simulink model "OREGO"  (Simulink 10.0)
settings: Solver=ode45  StartTime=0.0  StopTime=360  RelTol=1e-3  EnableMultiTasking=on
settings Model: Creator=UX31  LastModifiedBy=unknown
settings DataIOCC: LimitDataPoints=on
settings DebuggingCC: UnderspecifiedInitializationDetection=Simplified  MergeDetectMultiDrivingBlocksExec=error  SolverPrmCheckMsg=warning
settings GRTTargetCC: GeneratePreprocessorConditionals=Disable all  CombineOutputUpdateFcns=on  GRTInterface=off
settings ConfigComp: CovExternalEMLEnable=off  CovSFcnEnable=off

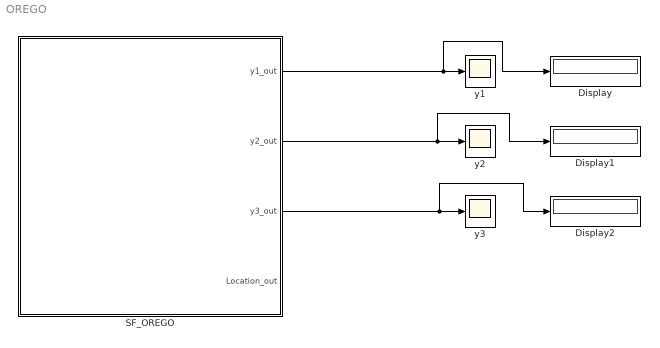
== system OREGO ==
  Display : Display
  Display1 : Display
  Display2 : Display
  SF_OREGO : Stateflow chart  TreatAsAtomicUnit=on
  y1 : Scope
  y2 : Scope
  y3 : Scope
  wires:
  SF_OREGO/1(y1_out) -> Display/1, y1/1
  SF_OREGO/2(y2_out) -> Display1/1, y2/1
  SF_OREGO/3(y3_out) -> Display2/1, y3/1

== stateflow chart SF_OREGO ==
  settings: updateMethod=CONTINUOUS
  state OREGO
    du:
    y1_dot=s*(y2-y1*y2+y1-q*y1^2);
    y2_dot=(1/s)*(0-y2-y1*y2+y3);
    y3_dot=w*(y1-y3);
    y1_out=y1;
    y2_out=y2;
    y3_out=y3;
    Location_out =1;
  (default) -> OREGO : {y1=1;y2=2;y3=3}
  data: y1 local double; y1_out output double; y2 local double; y2_out output double; y3 local double; y3_out output double; Location_out output double; s constant double =77.27; q constant double =8.375*10^-6; w constant double =0.161
  data y1 settings: updateMethod=SF_CONTINUOUS_TIME_DATA
  data y2 settings: updateMethod=SF_CONTINUOUS_TIME_DATA
  data y3 settings: updateMethod=SF_CONTINUOUS_TIME_DATA
